simulink model "LED_S_Comm"  (R2022b)
settings: Solver=FixedStepAuto  StartTime=0.0  StopTime=10.0  FixedStep=1e-3  RelTol=1e-3  EnableMultiTasking=on
libraries: frdmk64flib x5
settings Model: ExtModeTrigDuration=5  Creator=Ali Umar  LastModifiedBy=seankhaira
settings OptimizationCC: EnhancedBackFolding=on  PassReuseOutputArgsAs=Individual arguments  ZeroExternalMemoryAtStartup=off  ZeroInternalMemoryAtStartup=off  MaxStackSize=64  OptimizeBlockOrder=speed  DifferentSizesBufferReuse=on  OptimizationCustomize=off  EfficientTunableParamExpr=on
settings DebuggingCC: ParameterTunabilityLossMsg=error
settings HardwareCC: ProdBitPerPointer=32  ProdBitPerSizeT=32  ProdBitPerPtrDiffT=32  ProdLargestAtomicInteger=Long  ProdLargestAtomicFloat=Double  ProdWordSize=32  ProdHWDeviceType=ARM Compatible->ARM Cortex
settings SFSimCC: MATLABDynamicMemAlloc=off
settings RTWCC: Description=Embedded Coder  SystemTargetFile=ert.tlc  HardwareBoard=NXP FRDM-K64F  TLCOptions="-aInlineSetEventsForThisBaseRateFcn=TLC_FALSE -aSuppressMultiTaskScheduler=TLC_FALSE  -aRateBasedStepFcn=0"  TemplateMakefile=ert_default_tmf  Toolchain=GNU Tools for ARM Embedded Processors
settings CodeAppCC: ForceParamTrailComments=on  IgnoreCustomStorageClasses=off  OperatorAnnotations=on  SimulinkDataObjDesc=on  SFDataObjDesc=on  InsertBlockDesc=on
settings ERTTargetCC: ExtModeTransport=4  ExtModeMexFile=sendToCommService

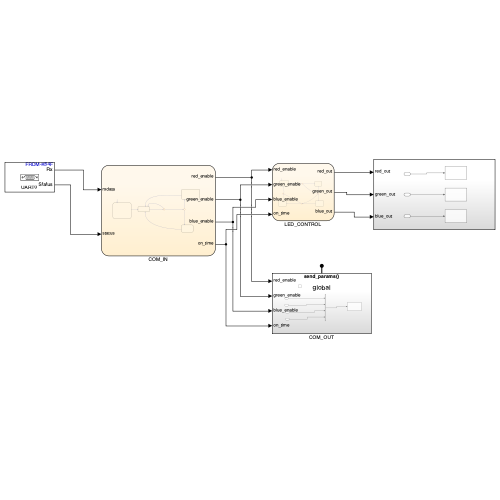
[thumbnail: Simulink's stored preview of the top-level diagram]
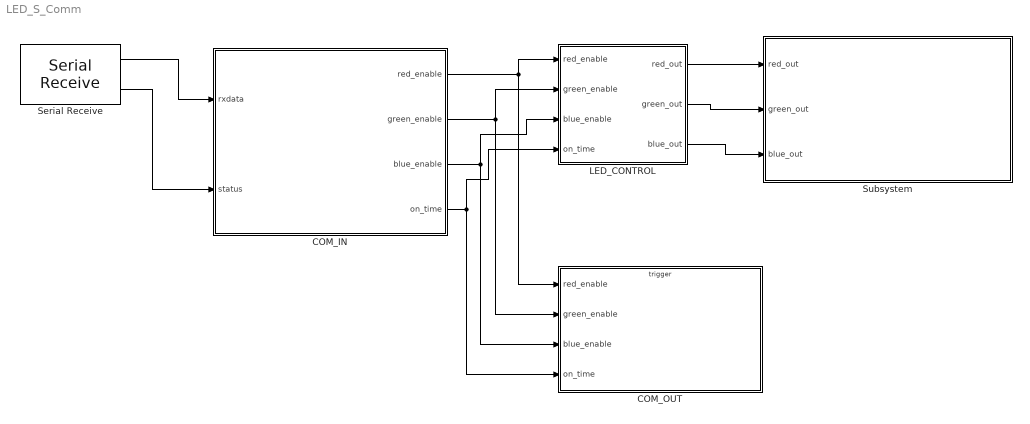
== system LED_S_Comm ==
  COM_IN : Stateflow chart  TreatAsAtomicUnit=on
  COM_OUT : Subsystem  TreatAsAtomicUnit=on
  LED_CONTROL : Stateflow chart  TreatAsAtomicUnit=on
  Serial Receive : frdmk64flib/Serial Receive  SCIModule=0  Baudrate=uint32(9600)  Parity=None  StopBits=1  HardwareFlowControl=None  ByteOrder=LittleEndian  DataType=uint8  DataLength=6  BlockingMode=off  OutputStatus=on  SampleTime=-1
  Subsystem : Subsystem
  wires:
  LED_CONTROL/2(green_out) -> Subsystem/2(green_out)
  COM_IN/2(green_enable) -> LED_CONTROL/2(green_enable), COM_OUT/2(green_enable)
  COM_IN/4(on_time) -> LED_CONTROL/4(on_time), COM_OUT/4(on_time)
  LED_CONTROL/3(blue_out) -> Subsystem/3(blue_out)
  COM_IN/1(red_enable) -> LED_CONTROL/1(red_enable), COM_OUT/1(red_enable)
  LED_CONTROL/1(red_out) -> Subsystem/1(red_out)
  COM_IN/3(blue_enable) -> LED_CONTROL/3(blue_enable), COM_OUT/3(blue_enable)
  Serial Receive/1 -> COM_IN/1(rxdata)
  Serial Receive/2 -> COM_IN/2(status)

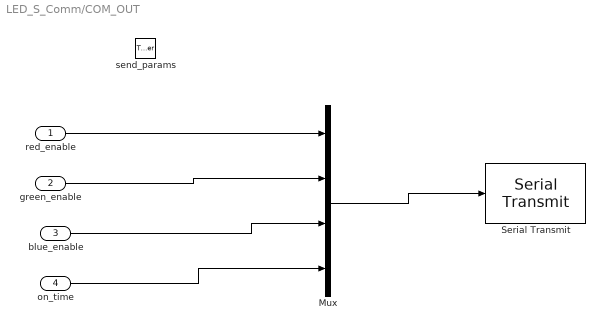
== system LED_S_Comm/COM_OUT ==
  red_enable : Inport
  green_enable : Inport  Port=2
  blue_enable : Inport  Port=3
  on_time : Inport  Port=4
  send_params : TriggerPort  TriggerType=function-call  IsSimulinkFunction=on  FunctionName=send_params  VariantControl=(inherit)
  Mux : Mux
  Serial Transmit : frdmk64flib/Serial Transmit  SCIModule=0  Baudrate=uint32(9600)  Parity=None  StopBits=1  HardwareFlowControl=None  ByteOrder=LittleEndian  BlockingMode=on  OutputStatus=off
  wires:
  red_enable/1 -> Mux/1
  green_enable/1 -> Mux/2
  blue_enable/1 -> Mux/3
  on_time/1 -> Mux/4
  Mux/1 -> Serial Transmit/1

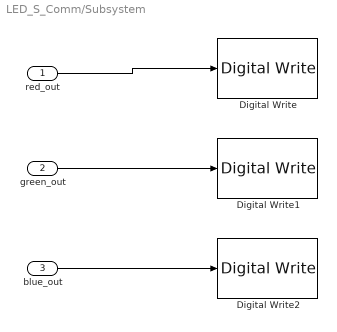
== system LED_S_Comm/Subsystem ==
  red_out : Inport
  green_out : Inport  Port=2
  blue_out : Inport  Port=3
  Digital Write : frdmk64flib/Digital Write  Whichpin=RED_LED
  Digital Write1 : frdmk64flib/Digital Write  Whichpin=GREEN_LED
  Digital Write2 : frdmk64flib/Digital Write  Whichpin=BLUE_LED
  wires:
  green_out/1 -> Digital Write1/1
  red_out/1 -> Digital Write/1
  blue_out/1 -> Digital Write2/1

== stateflow chart LED_S_Comm/LED_CONTROL ==
  state OFF
    entry:
    red_out = 0;
    green_out = 0;
    blue_out = 0;
  state RED_ON
    entry:
    red_out = 1;
    green_out = 0;
    blue_out = 0;
  state BLUE_ON
    entry:
    red_out = 0;
    green_out = 0;
    blue_out = 1;
  state GREEN_ON
    entry:
    red_out = 0;
    green_out = 1;
    blue_out = 0;
  (default) -> OFF
  OFF -> (junction 3) : after(on_time,sec)
  (junction 3) -> RED_ON [order 1] : [red_enable == 1]
  (junction 3) -> (junction 8) [order 2]
  RED_ON -> (junction 8) : after(on_time,sec)
  (junction 16) -> OFF
  (junction 12) -> (junction 16) [order 2]
  (junction 8) -> (junction 12) [order 2]
  BLUE_ON -> (junction 16) : after(on_time,sec)
  (junction 8) -> GREEN_ON [order 1] : [green_enable == 1]
  (junction 12) -> BLUE_ON [order 1] : [blue_enable == 1]
  GREEN_ON -> (junction 12) : after(on_time,sec)
  data: red_enable input; green_enable input; blue_enable input; on_time input; red_out output; green_out output; blue_out output

== stateflow chart LED_S_Comm/COM_IN ==
  settings: executeAtInitialization=1
  state SET_PARAM
    entry:
    red_enable = rxdata(3);
    green_enable = rxdata(4);
    blue_enable = rxdata(5);
    on_time = rxdata(6);
  state INITIAL
    %set initial parameters
    entry:
    red_enable = 0;
    green_enable = 0;
    blue_enable = 0;
    on_time = 1; %seconds
  state STANDBY
    %wait for com
  state ECHO_PARAM
    entry:
    send_params();
  SET_PARAM -> STANDBY
  (default) -> INITIAL
  (junction 21) -> SET_PARAM [order 1] : [rxdata(2)== hex2dec('55')]
  (junction 18) -> STANDBY [order 2]
  INITIAL -> STANDBY
  STANDBY -> (junction 18) : [status==0]
  (junction 18) -> (junction 21) [order 1] : [rxdata(1)== hex2dec('16')]
  (junction 21) -> ECHO_PARAM [order 2] : [rxdata(2)== hex2dec('22')]
  ECHO_PARAM -> STANDBY
  data: rxdata input; status input; red_enable output uint8; green_enable output uint8; blue_enable output uint8; on_time output uint8
